simulink library "dspsrcs2"  (Simulink 4.00)
values from neighbouring files (symbols this model uses):
  beta = varargin{4}; if isempty(beta), beta=5; end    [dspwdes.m]
  c = []    [dspfdes.m]    (also in liblinks.m = cell2struct(v,f,1); sbufscop.m = 'auto')
  p = {'Units','Position'}    [sdspfscope.m]    (also in sdspfscope2.m = get(hax(numAxes),'pos'); sdspmview.m; sdspmview2.m; sdspwfall.m = feval(printFcn,newfig))
undefined symbols (not defined in the file or in its folder): bps, deviceID, fSize, High, nChans, qSize, sRate
libraries: dspmtrx2 x3, dspswit2 x2, dspbdsp2 x1
settings Model: Creator=lelas  LastModifiedBy=rajbabu

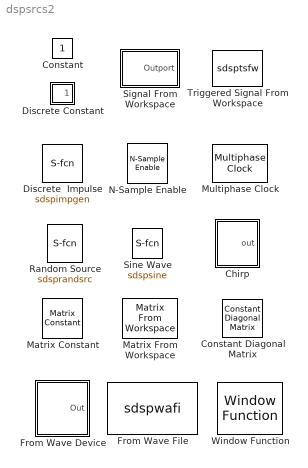
== system dspsrcs2 ==
  Chirp : Subsystem  mask(Chirp){method=Linear, f0=0.1, t1=1, f1=10, phi=0}
      mask prompts: method "Frequency sweep:"; f0 "Initial frequency (Hz):"; t1 "Target time (secs):"; f1 "Frequency at target time (Hz):"; phi "Initial phase (degrees):"
      mask help: Generate swept-frequency cosine with specified instantaneous frequency trajectory.
      mask init:
      | [t,y,txt] = dspblkchirp('icon');
      | [beta,p] = dspblkchirp('param',method,f0,f1,t1);
      settings: RTWFcnNameOpts=Auto  RTWFileNameOpts=Auto
      mask Help: web(dspbhelp);
      mask StyleString: popup(Linear|Quadratic|Logarithmic),edit,edit,edit,edit
      mask Display:
      | plot(t,y);
      | text(.2,.85,txt)
  Constant : Constant  Value=1
  Constant Diagonal Matrix : dspmtrx2/Constant Diagonal Matrix  n=3  q=1
  Discrete Constant : Subsystem  mask(Discrete Constant){Value=1, Ts=1}
      mask prompts: Value "Constant value:"; Ts "Sample time:"
      mask help: Output a discrete-time constant.
      settings: RTWFcnNameOpts=Auto  RTWFileNameOpts=Auto
      mask Help: web(dspbhelp);
      mask Display: disp(&1);
  Discrete  Impulse : S-Function  FunctionName=sdspimpgen  Parameters=Delay, SampleTime,FrameSample,Datatype  PortCounts=[]  SFunctionModules=''  mask(Discrete Impulse ){Delay=0, SampleTime=1, FrameSample=1, Datatype=Double}
      mask prompts: SampleTime "Sample time:"; FrameSample "Samples per frame:"; Datatype "Data type:"
      mask help: Output a discrete unit impulse. The impulse will be offset by the number of samples in the Delay parameter.
      mask init:
      | [x,y]=dspblkimpgen;
      mask Help: web(dspbhelp);
      mask StyleString: edit,edit,edit,popup(Double|Single|Boolean)
      mask Display: plot(x,y)
  From Wave Device : Subsystem  mask(From Wave Device){SampleRate=8000, UserRate=16000, SampleWidth=16, Stereo=off, SamplesPerFrame=512, QueueDuration=3, useDefaultDevice=on, userDeviceID=1}
      mask prompts: SampleRate "Sample rate (Hz):"; UserRate "User-defined sample rate (Hz):"; SampleWidth "Sample width (bits):"; SamplesPerFrame "Samples per frame:"; QueueDuration "Queue duration (seconds):"; useDefaultDevice "Use default audio device"; userDeviceID "Audio device ID: (1=1st device, 2=2nd device, ...)"
      mask help: Reads audio data samples from a standard Windows audio device in real time. Only for Win95/98/NT.
      mask init:
      | [x,y,x1,y1,x2,y2] = dspblkwai('icon');
      | [nChans, sRate, bps, fSize, qSize, deviceID] = dspblkwai('init', ...
      |              UserRate,SamplesPerFrame,QueueDuration, userDeviceID);
      settings: RTWFcnNameOpts=Auto  RTWFileNameOpts=Auto
      mask Help: web(dspbhelp);
      mask StyleString: popup(8000|11025|22050|44100|User-defined),edit,popup(8|16),checkbox,edit,edit,checkbox,edit
      mask CallbackString: dspblkwai;||||||dspblkwai;|
      mask Display:
      | patch(x1,y1); patch(x,y,[1 1 1]*.5);
      | patch(x2,y2);
      | plot(-.4,0,1.4,2)
  From Wave File : S-Function  FunctionName=sdspwafi  Parameters=fName, SampleRate, NChannels, SamplesPerFrame  PortCounts=[]  SFunctionModules=winmm.lib  mask(From Wave File){FileName=c:\winnt\media\chimes, SamplesPerFrame=256}
      mask prompts: FileName "File name:"; SamplesPerFrame "Samples per frame:"
      mask help: Reads audio data samples from a standard Windows PCM format ".WAV" audio file. Only for Win95/98/NT.
      mask init:
      | [fName,dName,SampleRate,NChannels,mode,err] = dspblkwafi('init');
      | if ~isempty(err), error(err); end
      mask Help: web(dspbhelp);
      mask Display: disp(['From Wave File\n' dName '\n' mode]);
  Matrix Constant : dspmtrx2/Matrix Constant  M=rand(3,3)
  Matrix From Workspace : dspmtrx2/Matrix From Workspace  U=rand(3,3,5)  Ts=1
  Multiphase Clock : dspswit2/Multiphase Clock  ClkFreq=1  NumPhases=4  StartPhase=1  DutyCycle=3  ActiveLevel=High (1)
  N-Sample Enable : dspswit2/N-Sample Enable  N=8  ActiveLevel=High (1)  reset=off  TriggerType=rising  Ts=1
  Random Source : S-Function  FunctionName=sdsprandsrc  Parameters=SrcType,Min,Max,Mean,Var,Seed,Inherit,SampMode,SampTime,SampFrame,OutComplex  PortCounts=[]  SFunctionModules=''  mask(Random Source){SrcType=Uniform, Min=0, Max=1, Mean=0, Var=1, Seed=1, Inherit=off, SampMode=Discrete, SampTime=1, SampFrame=1, OutComplex=Real}
      mask prompts: SrcType "Source type:"; Min "Minimum:"; Max "Maximum:"; Var "Variance:"; Seed "Initial seed:"; Inherit "Inherit output port attributes"; SampMode "Sample mode:"; SampTime "Sample time:"; SampFrame "Samples per frame:"; OutComplex "Output complexity:"
      mask help: Output a uniformly or Gaussian (normally) distributed random signal. Output is repeatable for a given seed.
      mask init:
      | [x,y]=dspblkrandsrc;
      mask Help: web(dspbhelp);
      mask StyleString: popup(Uniform|Gaussian),edit,edit,edit,edit,edit,checkbox,popup(Continuous|Discrete),edit,edit,popup(Real|Complex)
      mask CallbackString: dspblkrandsrc;||||||dspblkrandsrc;|dspblkrandsrc;|||
      mask Display: plot(x,y);
  Signal From Workspace : Subsystem  mask(Signal From Workspace){X=1:10, Ts=1, nsamps=1}
      mask prompts: X "Signal:"; Ts "Sample time:"; nsamps "Samples per frame:"
      mask help:
      | Output successive signal samples obtained from the MATLAB workspace at each sample time.
      |
      | A signal matrix is interpreted as having one channel per column.  Signal columns may be buffered into frames by specifying a number of samples per frame greater than 1.
      mask init:
      | [s,Ts] = dspblksfw('init', X,Ts,nsamps);
      settings: RTWFcnNameOpts=Auto  RTWFileNameOpts=Auto
      mask Help: web(dspbhelp);
      mask Display: disp(&1)
  Sine Wave : S-Function  FunctionName=sdspsine  Parameters=Amplitude,Frequency,Phase,SampleMode,OutComplex,CompMethod,SampleTime,SamplesPerFrame,ResetState  PortCounts=[]  SFunctionModules=''  mask(Sine Wave){Amplitude=1, Frequency=100, Phase=0, SampleMode=Discrete, OutComplex=Real, CompMethod=Trigonometric Fcn, SampleTime=1/1000, SamplesPerFrame=1, ResetState=Restart at time zero}
      mask prompts: Frequency "Frequency (Hz):"; Phase "Phase (rads):"; SampleMode "Sample mode:"; OutComplex "Output complexity:"; CompMethod "Computation method:"; SampleTime "Sample time:"; SamplesPerFrame "Samples per frame:"; ResetState "State when re-enabled:"
      mask help: Output samples of a sinusoid. More than one sinusoid may be generated simultaneously by entering a vector of values for the amplitude, frequency, and/or phase.
      mask init:
      | [x,y] = dspblksine('icon');
      mask Help: web(dspbhelp);
      mask StyleString: edit,edit,edit,popup(Continuous|Discrete),popup(Real|Complex),popup(Trigonometric Fcn|Table Lookup|Differential),edit,edit,popup(Restart at time zero|Catch up to simulation time)
      mask CallbackString: |||dspblksine;|dspblksine;|dspblksine;|||
      mask Display: plot(x,y)
  Triggered Signal From Workspace : S-Function  FunctionName=sdsptsfw  Parameters=U,cyclic,ic,trigtype,nsamps  PortCounts=[]  SFunctionModules=''  mask(Triggered Signal From Workspace){X=1:10, trigtype=Rising edge, cyclic=off, ic=0, nsamps=1}
      mask prompts: X "Signal:"; trigtype "Trigger type:"; cyclic "Output signal repeatedly"; ic "Initial output:"; nsamps "Samples per frame:"
      mask help:
      | Output successive signal samples obtained from the MATLAB workspace when a trigger event occurs.
      |
      | A signal matrix is interpreted as having one channel per column.  Signal columns may be buffered into frames by specifying a number of samples per frame greater than 1.
      mask init:
      | X = double(X);
      | [x,y]=dspblktsfw('icon',trigtype);
      | U = dspblktsfw('init', X,nsamps);
      | ic = double(ic);
      mask Help: web(dspbhelp);
      mask StyleString: edit,popup(Rising edge|Falling edge|Either edge),checkbox,edit,edit
      mask Display: plot(x,y); disp(&1);
  Window Function : dspbdsp2/Window Function  winmode=Generate window  wintype=Hamming  N=64  Rs=50  beta=10  winsamp=Symmetric  NChans=1

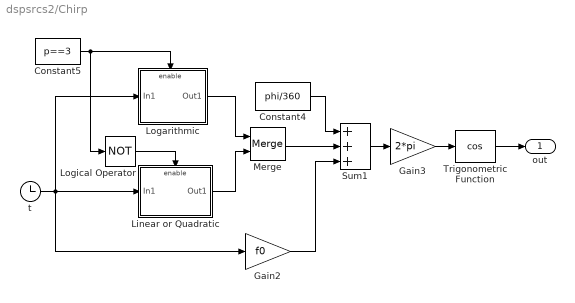
== system dspsrcs2/Chirp ==
  Constant4 : Constant  Value=phi/360
  Constant5 : Constant  Value=p==3
  Gain2 : Gain  Gain=f0  Multiplication=Element-wise(K.*u)  SaturateOnIntegerOverflow=on
  Gain3 : Gain  Gain=2*pi  Multiplication=Element-wise(K.*u)  SaturateOnIntegerOverflow=on
  Linear or Quadratic : Subsystem  TreatAsAtomicUnit=on
      settings: RTWFcnNameOpts=Auto  RTWFileNameOpts=Auto
  Logarithmic : Subsystem  TreatAsAtomicUnit=on
      settings: RTWFcnNameOpts=Auto  RTWFileNameOpts=Auto
  Logical Operator : Logic  Operator=NOT  Inputs=1
  Merge : Merge  Inputs=2  AllowUnequalInputPortWidths=off  InputPortOffsets=[]
  Sum1 : Sum  Inputs=3  SaturateOnIntegerOverflow=on
  Trigonometric Function : Trigonometry  Operator=cos  OutputSignalType=auto
  t : Clock
      settings: DisplayTime=off
  out : Outport  Port=1
  wires:
  Constant5/1 -> Logical Operator/1, Logarithmic/Enable
  Trigonometric Function/1 -> out/1
  Gain3/1 -> Trigonometric Function/1
  Sum1/1 -> Gain3/1
  Constant4/1 -> Sum1/1
  Merge/1 -> Sum1/2
  Gain2/1 -> Sum1/3
  Logarithmic/1(Out1) -> Merge/1
  Linear or Quadratic/1(Out1) -> Merge/2
  t/1 -> Gain2/1, Logarithmic/1(In1), Linear or Quadratic/1(In1)
  Logical Operator/1 -> Linear or Quadratic/Enable

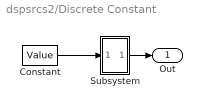
== system dspsrcs2/Discrete Constant ==
  Constant : Constant  Value=Value
  Subsystem : Subsystem
      settings: RTWFcnNameOpts=Auto  RTWFileNameOpts=Auto
  Out : Outport  Port=1
  wires:
  Subsystem/1(Out) -> Out/1
  Constant/1 -> Subsystem/1(In1)

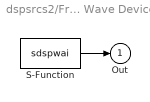
== system dspsrcs2/From Wave Device ==
  S-Function : S-Function  FunctionName=sdspwai  Parameters=nChans,sRate,bps,fSize,qSize,deviceID  PortCounts=[]  SFunctionModules=winmm.lib
  Out : Outport  Port=1  InitialOutput=0
  wires:
  S-Function/1 -> Out/1

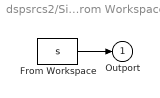
== system dspsrcs2/Signal From Workspace ==
  From Workspace : FromWorkspace  VariableName=s  SampleTime=Ts  Interpolate=off  OutputAfterFinalValue=SettingToZero
  Outport : Outport  Port=1  InitialOutput=0
  wires:
  From Workspace/1 -> Outport/1

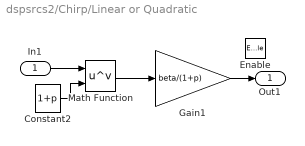
== system dspsrcs2/Chirp/Linear or Quadratic ==
  In1 : Inport  Port=1
  Enable : EnablePort
  Constant2 : Constant  Value=1+p
  Gain1 : Gain  Gain=beta/(1+p)  Multiplication=Element-wise(K.*u)  SaturateOnIntegerOverflow=on
  Math Function : Math  Operator=pow  OutputSignalType=auto
  Out1 : Outport  Port=1  InitialOutput=0
  wires:
  Constant2/1 -> Math Function/2
  Math Function/1 -> Gain1/1
  In1/1 -> Math Function/1
  Gain1/1 -> Out1/1

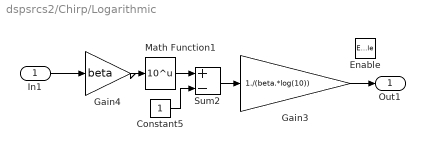
== system dspsrcs2/Chirp/Logarithmic ==
  In1 : Inport  Port=1
  Enable : EnablePort
  Constant5 : Constant  Value=1
  Gain3 : Gain  Gain=1./(beta.*log(10))  Multiplication=Element-wise(K.*u)  SaturateOnIntegerOverflow=on
  Gain4 : Gain  Gain=beta  Multiplication=Element-wise(K.*u)  SaturateOnIntegerOverflow=on
  Math Function1 : Math  Operator=10^u  OutputSignalType=auto
  Sum2 : Sum  Inputs=+-  SaturateOnIntegerOverflow=on
  Out1 : Outport  Port=1  InitialOutput=0
  wires:
  In1/1 -> Gain4/1
  Math Function1/1 -> Sum2/1
  Sum2/1 -> Gain3/1
  Constant5/1 -> Sum2/2
  Gain4/1 -> Math Function1/1
  Gain3/1 -> Out1/1

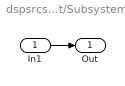
== system dspsrcs2/Discrete Constant/Subsystem ==
  In1 : Inport  Port=1  SampleTime=Ts
  Out : Outport  Port=1
  wires:
  In1/1 -> Out/1
